simulink model "aula1_R2015"  (R2015a)
settings: Solver=ode3  StartTime=0.0  StopTime=2  RelTol=1e-3
values from neighbouring files (symbols this model uses):
  wn = 10    [aula1_teste.m]
settings Model: CovModelRefEnable=off  Creator=CBA2016-05  LastModifiedBy=CBA2016-05
settings DataIOCC: LimitDataPoints=off  SaveFormat=Dataset
settings HardwareCC: ProdBitPerPointer=64  ProdLargestAtomicFloat=Float  ProdIntDivRoundTo=Zero  ProdEndianess=LittleEndian  ProdHWDeviceType=Specified
settings ModelReferenceCC: PropagateSignalLabelsOutOfModel=on

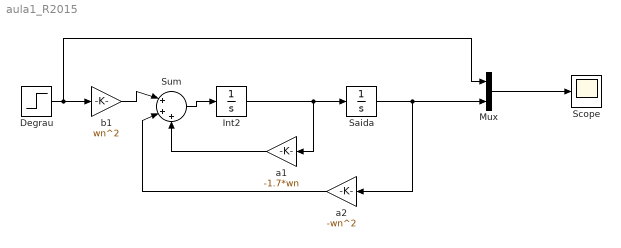
== system aula1_R2015 ==
  Degrau : Step  Time=0  SampleTime=0
  Int2 : Integrator
  Mux : Mux  Inputs=2
  Saida : Integrator
  Scope : Scope
      settings: TimeRange=auto  MaxDataPoints=5000  SaveName=X  YMin=-0.12582  YMax=1.13234  SampleTime=-1  DataFormat=Array
  Sum : Sum  Inputs=|+++
  a1 : Gain  Gain=-1.7*wn
  a2 : Gain  Gain=-wn^2
  b1 : Gain  Gain=wn^2
  wires:
  Int2/1 -> a1/1, Saida/1
  Mux/1 -> Scope/1
  Saida/1 -> a2/1, Mux/2
  b1/1 -> Sum/1
  Degrau/1 -> Mux/1, b1/1
  Sum/1 -> Int2/1
  a1/1 -> Sum/3
  a2/1 -> Sum/2
